simulink model "sldemo_tableplot"  (Simulink 7.6)
settings: Solver=ode2  SolverMode=SingleTasking  StartTime=0.0  StopTime=22  FixedStep=.008  RelTol=1e-3
PreLoadFcn:
  | load sldemo_tableplot_data;
  | tabfig = figure;
  | hda = daexplr;
  | set(hda, 'position', [6 458 1077 544] );
  | set( tabfig, 'Position', [550, 415, 674, 510] );
InitFcn:
  | mh = get_param('sldemo_tableplot','object');
  | luth = get_param('sldemo_tableplot/Look-Up Table (n-D)','object');
  | hda.view(mh);
  | hda.view(luth);
StopFcn:
  | sldemo_tableplot_comet(luth,logsOut);
undefined symbols (not defined in the file or in its folder): one, two
Description:
  | Interpolation Algorithm Selection and Trajectory Animation
  | 
  | This model employs a dynamic comet plot to visualize the result of changing
  | the interpolation and extrapolation options for a 2-D data set running in a
  | Lookup Table n-D block.  Algorithm options can be employed in different
  | situations to tradeoff accuracy, smoothness, data size, and performance.
  | 
  | Try opening the model and using the lookup table block's dialog to
  | change the interpolation and extrapolation algorithms. A copy of the
  | dialog is embedded in the right hand pane in the  Model Explorer and
  | will show up after the first simulation.  The Model Explorer is a
  | new component in Simulink(R) 6.0.  You can enter and tweak values for
  | the entire model and its blocks from the Model Explorer, including settings
  | for model configuration parameters, Simulink blocks, Stateflow(R) charts, and
  | Real-Time Workshop(R) settings for code generation and data management.
  | 
  | To make the plot, data from the simulation is logged using the non-intrusive
  | logging features in Simulink 6.0.  Non-intrusive logging is annotated on the
  | block diagram by the small blue "transmitter antennas" on certain block output
  | ports. These logging points can be set from the MATLAB(R) command line using
  | set_param(), or via the Signal & Scope Manager from the Tools menu or the signal
  | properties dialog.
CloseFcn:
  | if exist('hda')
  |   hide(hda);
  |   clear('hda');
  | end
  | if exist('tabfig')
  |   if ishghandle(tabfig, 'figure')
  |       close(tabfig);
  |   end
  |   clear('tabfig');
  | end
  | clear('luth');
settings Model: Creator=The MathWorks Inc.  ExtModeTrigMode=oneshot  ExtModeArmWhenConnect=off  ExtModeAutoUpdateStatusClock=off
settings DataIOCC: LimitDataPoints=off  SaveOutput=off  SaveTime=off  SignalLoggingName=logsOut
settings OptimizationCC: BlockReduction=off  BooleanDataType=off  InlineInvariantSignals=on  InitFltsAndDblsToZero=on
settings DebuggingCC: SaveWithParameterizedLinksMsg=none  CheckExecutionContextPreStartOutputMsg=on  CheckExecutionContextRuntimeOutputMsg=on  SignalResolutionControl=TryResolveAllWithWarning  SolverPrmCheckMsg=none  MultiTaskDSMMsg=warning  MultiTaskCondExecSysMsg=none  SigSpecEnsureSampleTimeMsg=none
settings HardwareCC: TargetUnknown=on
settings RTWCC: IncludeERTFirstTime=on
settings GRTTargetCC: TargetFcnLib=ansi_tfl_tmw.mat

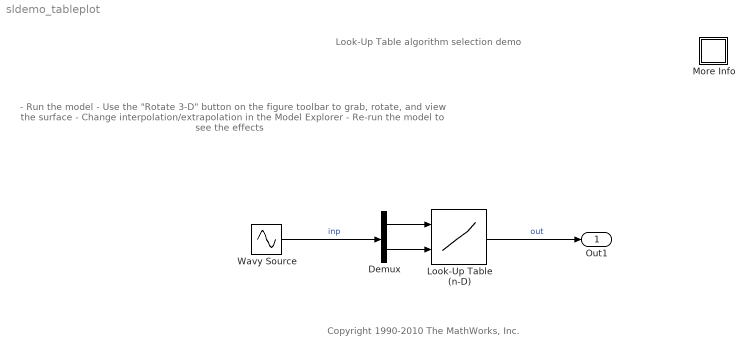
== system sldemo_tableplot ==
  note: - Run the model
      | - Use the "Rotate 3-D" button on the figure toolbar
      |   to grab, rotate, and view the surface
      | - Change interpolation/extrapolation in the Model Explorer
      | - Re-run the model to see the effects
  note: Look-Up Table algorithm selection demo
  note: Copyright 1990-2010 The MathWorks, Inc.
  Demux : Demux  Outputs=2
  Look-Up Table (n-D) : Lookup_n-D  BreakpointsForDimension1=one  BreakpointsForDimension2=two  Table=tab'  InputSameDT=on
      settings: AttributesFormatString=interpolation: %<interpMethod>\nextrapolation: %<extrapMethod>
  More Info : Subsystem
      settings: OpenFcn=showdemo(bdroot(gcb))
      mask Display: disp('?')
  Wavy Source : Sin  Amplitude=[22.5, 25]  Bias=[22.5, 45]  Frequency=[1.714, 1]  Phase=[pi, 0]  SampleTime=0
  Out1 : Outport
  wires:
  Look-Up Table (n-D)/1 -> Out1/1  "out"
  Wavy Source/1 -> Demux/1  "inp"
  Demux/1 -> Look-Up Table (n-D)/1
  Demux/2 -> Look-Up Table (n-D)/2

== system sldemo_tableplot/More Info ==
